simulink model "GFLIB_Limit_BAM"  (Simulink 9.3)
settings: Solver=VariableStepAuto  StartTime=0.0  StopTime=10.0  RelTol=1e-3
settings Model: Creator=nxa18952  LastModifiedBy=nxa18952
settings DataIOCC: SaveFormat=Dataset  SignalLoggingSaveFormat=Dataset  ReturnWorkspaceOutputs=on
settings OptimizationCC: LifeSpan=auto
settings DebuggingCC: UnderspecifiedInitializationDetection=Simplified  MergeDetectMultiDrivingBlocksExec=error  FcnCallInpInsideContextMsg=error  SFUnexpectedBacktrackingDiag=error  SFNoUnconditionalDefaultTransitionDiag=error  SFExecutionAtInitializationDiag=warning  ArithmeticOperatorsInVariantConditions=error
settings HardwareCC: ProdBitPerPointer=64  ProdBitPerSizeT=64  ProdBitPerPtrDiffT=64  ProdLargestAtomicFloat=Float  ProdIntDivRoundTo=Zero  ProdEndianess=LittleEndian  ProdWordSize=64  ProdHWDeviceType=Intel->x86-64 (Windows64)
settings ModelReferenceCC: PropagateSignalLabelsOutOfModel=on
settings SFSimCC: SimUseLocalCustomCode=on
settings RTWCC: RTWUseLocalCustomCode=on
settings CodeAppCC: StateflowObjectComments=off
settings GRTTargetCC: TargetLangStandard=C99 (ISO)  CombineOutputUpdateFcns=on  GRTInterface=off
settings ConfigComp: CovMetricSettings=dwe  CovHtmlReporting=off  CovSaveCumulativeToWorkspaceVar=off  CovSaveSingleToWorkspaceVar=off  CovExternalEMLEnable=on

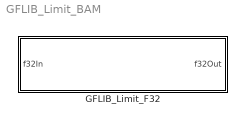
== system GFLIB_Limit_BAM ==
  GFLIB_Limit_F32 : Subsystem  TreatAsAtomicUnit=on  mask(GFLIB_Limit_F32){showStates=Hide (faster execution), f32LowerLimit=0, f32UpperLimit=0}
      mask prompts: showStates "Show internal states"; f32LowerLimit "f32LowerLimit (Lower limit)"; f32UpperLimit "f32UpperLimit (Upper limit)"
      mask help: Bit accurate model of GFLIB_Limit function in 32-bit fixed-point fractional implementation. Refer to the AMMCLIB User's Guide for further details.
      mask init:
      | if ~evalin('base','exist(''tS8'',''var'')')
      |   if (2 ~= exist('SWLIBS_Typedefs.mat','file'))
      |       error('File SWLIBS_Typedefs.mat is not on the Matlab path. Please add the AMMCLIB "bam" folder in the Matlab Search Path.');
      |   else
      |       evalin('base', 'load(''SWLIBS_Typedefs.mat'')');
      |   end
      | end
      | if showStates == 1
      |     % hidden state variables
      |     if strcmp(get_param([gcb '/f32LowerLimit'], 'BlockType'), 'Inport')
      |         posblk = get_param(gcb, 'Position');
      | 
      |         pos = get_param(    [gcb, '/f32LowerLimit'], 'Position');
      |         orient = get_param( [gcb, '/f32LowerLimit'], 'Orientation');
      |         delete_block(       [gcb, '/f32LowerLimit']);
      |         add_block('built-in/Ground', [gcb, '/f32LowerLimit'], 'Position', pos, 'Orientation', orient);
      | 
      |         pos = get_param(    [gcb, '/f32UpperLimit'], 'Position');
      |         orient = get_param( [gcb, '/f32UpperLimit'], 'Orientation');
      |         delete_block(       [gcb, '/f32UpperLimit']);
      |         add_block('built-in/Ground', [gcb, '/f32UpperLimit'], 'Position', pos, 'Orientation', orient);
      | 
      | 
      | 
      |         set_param([gcb '/f32In'], 'Port', '1');
      | 
      |         set_param([gcb '/f32Out'], 'Port', '1');
      | 
      |         set_param(gcb,'MaskEnables',{'on','on','on'});
      | 
      |         if (posblk(4) - posblk(2)) > 50
      |           height = 50;
      |           set_param(gcb,'Position',[posblk(1), posblk(2), posblk(3), posblk(2)+height])
      |         end
      |     end
      | else
      |     % shown state variables
      |     if strcmp(get_param([gcb '/f32LowerLimit'], 'BlockType'), 'Ground')
      |         posblk = get_param(gcb, 'Position');
      | 
      |         pos = get_param(    [gcb, '/f32LowerLimit'], 'Position');
      |         orient = get_param( [gcb, '/f32LowerLimit'], 'Orientation');
      |         delete_block(       [gcb, '/f32LowerLimit']);
      |         add_block('built-in/Inport', [gcb, '/f32LowerLimit'], 'Position', pos, 'Orientation', orient, 'OutDataTypeStr', 'int32');
      | 
      |         pos = get_param(    [gcb, '/f32UpperLimit'], 'Position');
      |         orient = get_param( [gcb, '/f32UpperLimit'], 'Orientation');
      |         delete_block(       [gcb, '/f32UpperLimit']);
      |         add_block('built-in/Inport', [gcb, '/f32UpperLimit'], 'Position', pos, 'Orientation', orient, 'OutDataTypeStr', 'int32');
      | 
      | 
      | 
      |         set_param([gcb '/f32In'], 'Port', '1');
      |         set_param([gcb '/f32LowerLimit'], 'Port', '2');
      |         set_param([gcb '/f32UpperLimit'], 'Port', '3');
      | 
      |         set_param([gcb '/f32Out'], 'Port', '1');
      | 
      |         set_param(gcb,'MaskEnables',{'on','off','off'});
      | 
      |         if (posblk(4) - posblk(2)) < 100
      |           height = 100;
      |           set_param(gcb,'Position',[posblk(1), posblk(2), posblk(3), posblk(2)+height])
      |         end
      |     end
      | end
      settings: RTWSystemCode=Inline
      mask TypeOptions showStates: Hide (faster execution) | Show (allows debugging; connect feedback loops manually)
      mask Callback showStates:
      | maskStr = get_param(gcb,'showStates');
      | if strcmp(maskStr,'Hide (faster execution)'),
      |     set_param(gcb,'MaskEnables',{'on','on','on'});
      | else
      |     set_param(gcb,'MaskEnables',{'on','off','off'});
      | end
      mask Display:
      | color('black');
      | pos = get_param(gcb, 'Position');
      | width = pos(3) - pos(1);
      | height = pos(4) - pos(2);
      | tX=width/2;
      | tY=height - 8;
      | color('black');
      | text(tX,tY, 'GFLIB_Limit_F32', 'horizontalAlignment', 'center');
      | if showStates == 2
      |   color('red');
      |   text(tX,tY - 20, ['debugging mode' char(13) char(10) '(limited performance)'], 'horizontalAlignment', 'center');
      | end

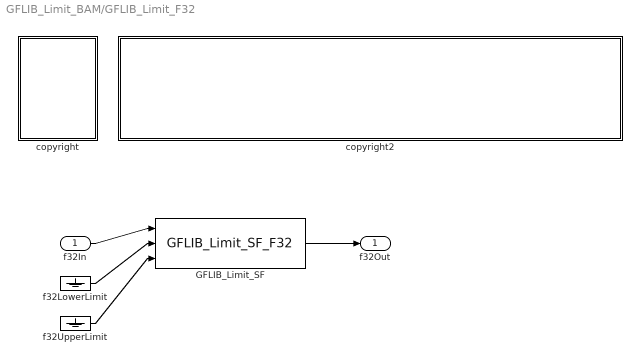
== system GFLIB_Limit_BAM/GFLIB_Limit_F32 ==
  f32In : Inport  OutDataTypeStr=int32
  GFLIB_Limit_SF : S-Function  FunctionName=GFLIB_Limit_SF_F32  Parameters=showStates,f32LowerLimit,f32UpperLimit  SFunctionDeploymentMode=off  EnableBusSupport=off
  copyright : Subsystem
      mask Display: text(10,90,'FILE:');text(10,75,'DESRIPTION:');text(10,60,'COPYRIGHT:');text(10,45,'VERSION:');text(10,30,'DATE:')
  copyright2 : Subsystem
      mask Display: text(10,90,'GFLIB_Limit_BAM_F32.mdl');text(10,75,'Limit function.');text(10,60,'NXP 2020');text(10,45,'1.0');text(10,30,'23-Mar-2020');
  f32LowerLimit : Ground
  f32UpperLimit : Ground
  f32Out : Outport
  wires:
  f32In/1 -> GFLIB_Limit_SF/1
  f32LowerLimit/1 -> GFLIB_Limit_SF/2
  f32UpperLimit/1 -> GFLIB_Limit_SF/3
  GFLIB_Limit_SF/1 -> f32Out/1

== system GFLIB_Limit_BAM/GFLIB_Limit_F32/copyright ==

== system GFLIB_Limit_BAM/GFLIB_Limit_F32/copyright2 ==
